simulink model "WithoutMOSFET"  (R2019b)
settings: Solver=VariableStepAuto  StartTime=0.0  StopTime=10.0  RelTol=1e-3
libraries: powerlib x10, simulink x6, pspsim x1
settings Model: Creator=ahmet  LastModifiedBy=ahmet

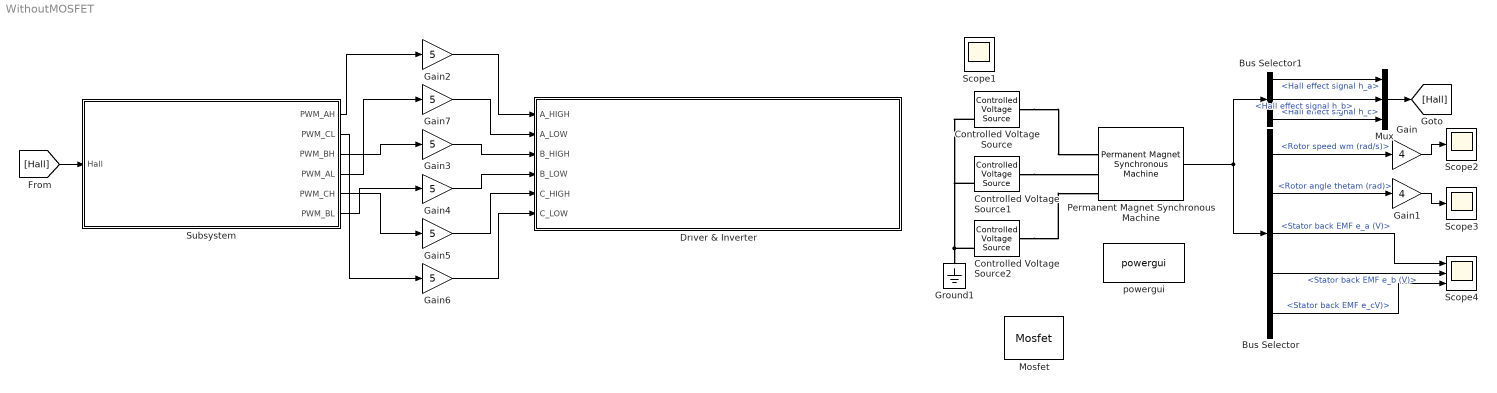
== system WithoutMOSFET ==
  Bus Selector : BusSelector  OutputSignals=Rotor speed wm (rad/s),Rotor angle thetam (rad),Stator back EMF e_a (V),Stator back EMF e_b (V),Stator back EMF e_cV)
  Bus Selector1 : BusSelector  OutputSignals=Hall effect signal h_a,Hall effect signal h_b,Hall effect signal h_c
  Controlled Voltage Source : powerlib/Electrical Sources/Controlled Voltage Source  Initialize=on  Source_Type=DC  Amplitude=0  Phase=0  Frequency=0  Measurements=None
      settings: SourceProductName=Simscape Electrical
  Controlled Voltage Source1 : powerlib/Electrical Sources/Controlled Voltage Source  Initialize=on  Source_Type=DC  Amplitude=0  Phase=0  Frequency=0  Measurements=None
      settings: SourceProductName=Simscape Electrical
  Controlled Voltage Source2 : powerlib/Electrical Sources/Controlled Voltage Source  Initialize=on  Source_Type=DC  Amplitude=0  Phase=0  Frequency=0  Measurements=None
      settings: SourceProductName=Simscape Electrical
  Drıver & Inverter : Subsystem
  Gain : Gain  Gain=4
  Gain1 : Gain  Gain=4
  Gain{2..7} (6 alike) : Gain  Gain=5
  Ground1 : powerlib/Elements/Ground  LConnTagsString=a
      settings: SourceProductName=Simscape Electrical
  Mosfet : powerlib/Power Electronics/Mosfet  Ron=0.1  Lon=0  Rd=0.01  Vfd=0  IC=0  Rs=1e5  Cs=inf  Measurements=on
      settings: SourceProductName=Simscape Electrical
  Mux : Mux  Inputs=3
  Permanent Magnet Synchronous Machine : powerlib/Machines/Permanent Magnet Synchronous Machine  NbPhases=3  FluxDistribution=Trapezoidal  RotorType=Round  MechanicalLoad=Torque Tm  PresetModel=No  ShowDetailedParameters=on  MeasurementBus=off  Resistance=2.8750  Inductance=8.5e-3  dqInductances=[8.5e-3, 8.5e-3]  La=0.000835  MachineConstant=Flux linkage established by magnets (V.s)  Flux=0.175  VoltageCst=146.6077  TorqueCst=1.4  Flat=120  Mechanical=[ 0.8e-3, 1e-3 4]  PolePairs=4  InitialConditions=[0,0, 0,0]  InitialConditions5ph=[0 0 0 0 0 0]  RefAngle=90 degrees behind phase A axis (modified Park)  IterativeDiscreteModel=Trapezoidal non iterative  TsBlock=-1  TsPowergui=0
  Scope1 : Scope  NumInputPorts=3
  Scope2 : Scope
  Scope3 : Scope
  Scope4 : Scope  NumInputPorts=3
  Subsystem : Subsystem
  powergui : powerlib/powergui  Priority=1  SimulationMode=Discrete  SampleTime=50e-6  frequency=60  Iterations=50  frequencyindice=0  Pbase=100e6  ErrMax=1e-4  UnitsV=kV  UnitsW=MW  buscounter=0  FunctionMessages=off  echomessages=off  EnableUseOfTLC=off  CurrentSourceSwitches=off  DisableSnubberDevices=off  DisableRonSwitches=off  DisableVfSwitches=off  DisplayEquations=off  AutomaticDiscreteSolvers=on  SolverType=Tustin/Backward Euler (TBE)  Interpol=off  ExternalGateDelay=off  methode=off  Ts=100  x0status=blocks  SPID=on  SwTol=0  HookPort=off  NonlinearTolerance=1e-4  nMaxIteration=100  ContinueOnMaxIteration=off  RestoreLinks=warning  ResistiveCurrentMeasurement=off  Frange=[0:2:500]  Ylog=off  Xlog=on  ShowGrid=off  save=off  variable=ZData  structure=0  ZoomFFT=off  StartTime=0.0  cycles=1  DisplayStyle=1  fundamental=60  FreqAxis=off  MaxFrequency=1000  frequencyindicesteady=1  RmsSteady=1  display=off
      settings: SourceProductName=Simscape Electrical
  wires:
  ? -> Scope1/3, Controlled Voltage Source2/1
  ? -> Scope1/2, Controlled Voltage Source1/1
  Subsystem/6("PWM_BL ") -> Gain4/1
  Bus Selector/2 -> Gain1/1  "<Rotor angle thetam (rad)>"
  Bus Selector/1 -> Gain/1  "<Rotor speed wm (rad/s)>"
  Bus Selector1/3 -> Mux/3  "<Hall effect signal h_c>"
  Gain6/1 -> Drıver & Inverter/6("C_LOW ")
  Gain2/1 -> Drıver & Inverter/1("A_HIGH ")
  Gain3/1 -> Drıver & Inverter/3("B_HIGH ")
  Gain5/1 -> Drıver & Inverter/5("C_HIGH ")
  Bus Selector/3 -> Scope4/1  "<Stator back EMF e_a (V)>"
  Subsystem/3("PWM_BH ") -> Gain3/1
  ? -> Scope1/1, Controlled Voltage Source/1
  Bus Selector/5 -> Scope4/3  "<Stator back EMF e_cV)>"
  Bus Selector1/1 -> Mux/1  "<Hall effect signal h_a>"
  Gain/1 -> Scope2/1
  Bus Selector1/2 -> Mux/2  "<Hall effect signal h_b>"
  Subsystem/2(PWM_CL) -> Gain6/1
  [Hall] -> Subsystem/1("Hall ")
  Gain1/1 -> Scope3/1
  Subsystem/4("PWM_AL ") -> Gain7/1
  Subsystem/5("PWM_CH ") -> Gain5/1
  Mux/1 -> [Hall]
  Gain4/1 -> Drıver & Inverter/4("B_LOW ")
  Bus Selector/4 -> Scope4/2  "<Stator back EMF e_b (V)>"
  Permanent Magnet Synchronous Machine/1 -> Bus Selector1/1, Bus Selector/1
  Gain7/1 -> Drıver & Inverter/2("A_LOW ")
  Subsystem/1(PWM_AH) -> Gain2/1
  connections:
  Controlled Voltage Source2/LConn1 -- Ground1/LConn1 -- Controlled Voltage Source/LConn1 -- Controlled Voltage Source1/LConn1
  Controlled Voltage Source1/RConn1 -- Permanent Magnet Synchronous Machine/LConn2
  Controlled Voltage Source/RConn1 -- Permanent Magnet Synchronous Machine/LConn1
  Controlled Voltage Source2/RConn1 -- Permanent Magnet Synchronous Machine/LConn3

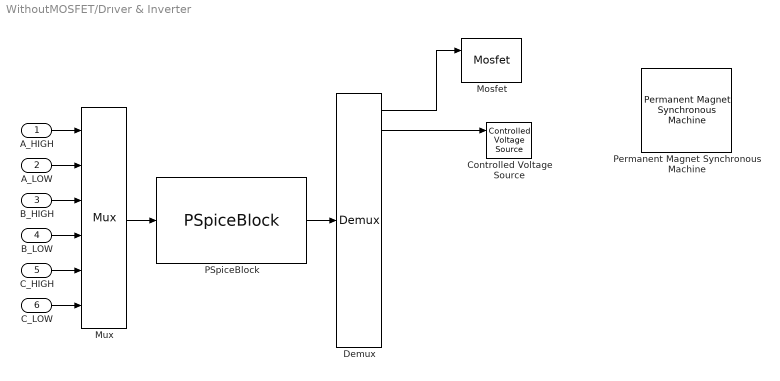
== system WithoutMOSFET/Drıver & Inverter ==
  "A_HIGH " : Inport
  "A_LOW " : Inport  Port=2
  "B_HIGH " : Inport  Port=3
  "B_LOW " : Inport  Port=4
  "C_HIGH " : Inport  Port=5
  "C_LOW " : Inport  Port=6
  Controlled Voltage Source : powerlib/Electrical Sources/Controlled Voltage Source  Initialize=on  Source_Type=DC  Amplitude=50  Phase=0  Frequency=0  Measurements=None
      settings: SourceProductName=Simscape Electrical
  Demux : Demux  Outputs=12
  Mosfet : powerlib/Power Electronics/Mosfet  Ron=0.1  Lon=0  Rd=0.01  Vfd=0  IC=0  Rs=1e5  Cs=inf  Measurements=on
      settings: SourceProductName=Simscape Electrical
  Mux : Mux  Inputs=6
      settings: DisplayOption=signals
  PSpiceBlock : pspsim/PSpiceBlock  SFunctionModules=''
      settings: SourceProductName=PSpice Block
  Permanent Magnet Synchronous Machine : powerlib/Machines/Permanent Magnet Synchronous Machine  NbPhases=3  FluxDistribution=Sinusoidal  RotorType=Round  MechanicalLoad=Torque Tm  PresetModel=No  ShowDetailedParameters=on  MeasurementBus=off  Resistance=0.0485  Inductance=8.5e-3  dqInductances=[8.5e-3,8.5e-3]  La=0.000395  MachineConstant=Flux linkage established by magnets (V.s)  Flux=0.1194  VoltageCst=86.6271  TorqueCst=0.7164  Flat=120  Mechanical=[0.0027 0.0004924 4 0]  PolePairs=4  InitialConditions=[0,0, 0,0]  InitialConditions5ph=[0 0 0 0 0 0]  RefAngle=90 degrees behind phase A axis (modified Park)  IterativeDiscreteModel=Trapezoidal non iterative  TsBlock=-1  TsPowergui=0
  wires:
  "B_LOW "/1 -> Mux/4
  "B_HIGH "/1 -> Mux/3
  "C_HIGH "/1 -> Mux/5
  "A_HIGH "/1 -> Mux/1
  "A_LOW "/1 -> Mux/2
  PSpiceBlock/1 -> Demux/1
  "C_LOW "/1 -> Mux/6
  Mux/1 -> PSpiceBlock/1
  Demux/1 -> Mosfet/1
  Demux/2 -> Controlled Voltage Source/1

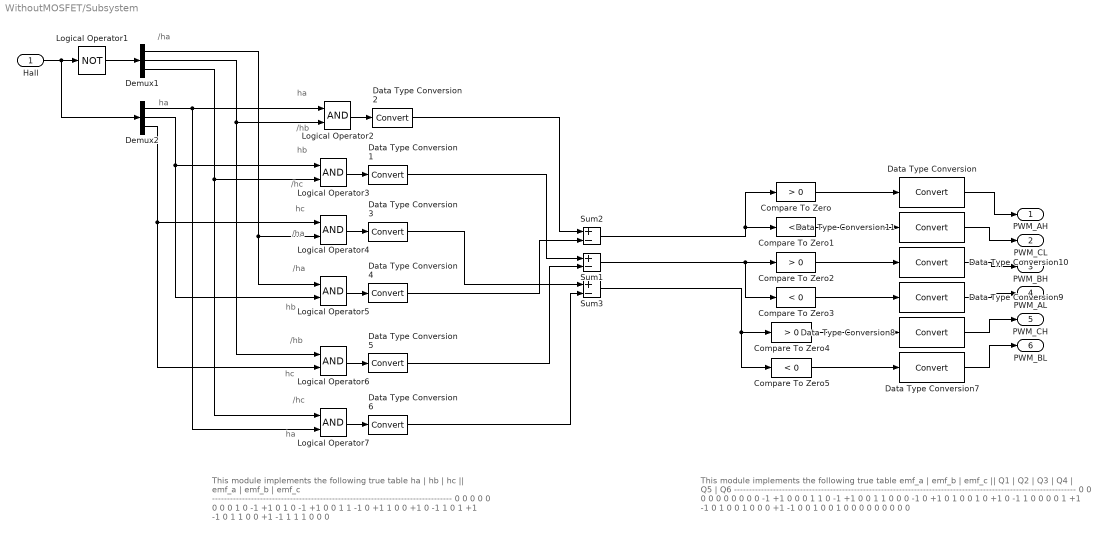
== system WithoutMOSFET/Subsystem ==
  note: hc
  note: /hc
  note: hb
  note: hc
  note: This module implements the following true table
      |
      |    ha   |   hb   |   hc   ||   emf_a   |   emf_b   |   emf_c
      |     --------------------------------------------------------------------------------
      | 0          0         0          0               0               0
      | 0          0         1          0               -1              +1
      | 0          1         0          -1              +1                0
      | 0          1         1          -1               0               +1
      | 1          0         0         +1               0               -1
      | 1          0         1         +1              -1                0
      | 1          1         0          0              +1               -1
      | 1          1         1          0               0                0
  note: ha
  note: /hb
  note: /hb
  note: /hc
  note: ha
  note: /ha
  note: ha
  note: hb
  note: /ha
  note: /ha
  note: This module implements the following true table
      |
      |    emf_a   |   emf_b   |   emf_c   ||   Q1   |   Q2   |   Q3   |   Q4   |   Q5   |   Q6
      |     ------------------------------------------------------------------------------------------------------------------
      |       0              0                0            0          0          0           0        0        0
      |       0               -1              +1          0          0          0           1        1        0
      |     -1              +1                0          0          1          1           0        0        0
      |     -1               0               +1          0          1         0           0        1        0
      |    +1               0                -1          1          0          0           0        0        1
      |    +1              -1                0           1          0          0           1        0        0
      |      0              +1               -1           0          0          1           0        0        1
      |     0              0                0             0          0          0           0        0        0
  "Hall " : Inport
  Compare To Zero : simulink/Logic and Bit Operations/Compare To Zero  relop=>  OutDataTypeStr=boolean  ZeroCross=off
  Compare To Zero1 : simulink/Logic and Bit Operations/Compare To Zero  relop=<  OutDataTypeStr=boolean  ZeroCross=off
  Compare To Zero2 : simulink/Logic and Bit Operations/Compare To Zero  relop=>  OutDataTypeStr=boolean  ZeroCross=off
  Compare To Zero3 : simulink/Logic and Bit Operations/Compare To Zero  relop=<  OutDataTypeStr=boolean  ZeroCross=off
  Compare To Zero4 : simulink/Logic and Bit Operations/Compare To Zero  relop=>  OutDataTypeStr=boolean  ZeroCross=off
  Compare To Zero5 : simulink/Logic and Bit Operations/Compare To Zero  relop=<  OutDataTypeStr=boolean  ZeroCross=off
  Data Type Conversion{,1..11} (12 alike) : DataTypeConversion
  Demux1 : Demux  Outputs=3
  Demux2 : Demux  Outputs=3
  Logical Operator1 : Logic  Operator=NOT  AllPortsSameDT=off  OutDataTypeStr=boolean
  Logical Operator{2..7} (6 alike) : Logic  AllPortsSameDT=off  OutDataTypeStr=boolean
  Sum1 : Sum  Inputs=+-  OutDataTypeStr=double
  Sum2 : Sum  Inputs=+-  OutDataTypeStr=double
  Sum3 : Sum  Inputs=+-  OutDataTypeStr=double
  PWM_AH : Outport
  PWM_CL : Outport  Port=2
  "PWM_BH " : Outport  Port=3
  "PWM_AL " : Outport  Port=4
  "PWM_CH " : Outport  Port=5
  "PWM_BL " : Outport  Port=6
  wires:
  Data Type Conversion6/1 -> Sum3/2
  Logical Operator2/1 -> Data Type Conversion2/1
  Logical Operator4/1 -> Data Type Conversion3/1
  Logical Operator3/1 -> Data Type Conversion1/1
  Demux2/2 -> Logical Operator3/1, Logical Operator5/2
  Demux1/2 -> Logical Operator2/2, Logical Operator6/1
  Logical Operator6/1 -> Data Type Conversion5/1
  Data Type Conversion3/1 -> Sum3/1
  Data Type Conversion1/1 -> Sum1/1
  Data Type Conversion5/1 -> Sum1/2
  Demux1/1 -> Logical Operator4/2, Logical Operator5/1
  Demux2/3 -> Logical Operator4/1, Logical Operator6/2
  Demux1/3 -> Logical Operator3/2, Logical Operator7/1
  Data Type Conversion4/1 -> Sum2/2
  Demux2/1 -> Logical Operator2/1, Logical Operator7/2
  "Hall "/1 -> Logical Operator1/1, Demux2/1
  Data Type Conversion2/1 -> Sum2/1
  Logical Operator5/1 -> Data Type Conversion4/1
  Logical Operator7/1 -> Data Type Conversion6/1
  Logical Operator1/1 -> Demux1/1
  Sum1/1 -> Compare To Zero2/1, Compare To Zero3/1
  Sum3/1 -> Compare To Zero4/1, Compare To Zero5/1
  Sum2/1 -> Compare To Zero/1, Compare To Zero1/1
  Compare To Zero/1 -> Data Type Conversion/1
  Data Type Conversion/1 -> PWM_AH/1
  Data Type Conversion7/1 -> "PWM_BL "/1
  Compare To Zero5/1 -> Data Type Conversion7/1
  Compare To Zero4/1 -> Data Type Conversion8/1
  Data Type Conversion8/1 -> "PWM_CH "/1
  Data Type Conversion9/1 -> "PWM_AL "/1
  Compare To Zero3/1 -> Data Type Conversion9/1
  Data Type Conversion10/1 -> "PWM_BH "/1
  Compare To Zero2/1 -> Data Type Conversion10/1
  Data Type Conversion11/1 -> PWM_CL/1
  Compare To Zero1/1 -> Data Type Conversion11/1
